simulink model "handsteuer_Joystick"  (Simulink 8.9)
settings: Solver=ode4  StartTime=0.0  StopTime=1200  FixedStep=0.01  RelTol=1e-3  EnableMultiTasking=on
undefined symbols (not defined in the file or in its folder): Joystick, National_Instruments, PCIe, Standard_Devices
libraries: sldrtlib x3, cstblocks x1
CloseFcn:
  | rtwprivate ssgencode ModelCloseRequest handsteuer_Joystick
settings Model: Creator=Praktikum  LastModifiedBy=prt01  SimulationMode=external  ExtModeTrigDuration=1000000
settings OptimizationCC: ExpressionDepthLimit=2147483647  InitFltsAndDblsToZero=on  LifeSpan=auto
settings DebuggingCC: SaveWithParameterizedLinksMsg=none  SignalResolutionControl=TryResolveAllWithWarning  SolverPrmCheckMsg=warning  MultiTaskDSMMsg=warning  MultiTaskCondExecSysMsg=none
settings HardwareCC: ProdBitPerPointer=64  ProdBitPerSizeT=64  ProdBitPerPtrDiffT=64  ProdLargestAtomicFloat=Float  ProdIntDivRoundTo=Zero  ProdEndianess=LittleEndian  ProdWordSize=64  ProdHWDeviceType=Intel->x86-64 (Windows64)
settings RTWCC: SystemTargetFile=sldrt.tlc  TemplateMakefile=sldrt.tmf  Description=Simulink Desktop Real-Time  RTWCompilerOptimization=on
settings CodeAppCC: MaxIdLength=95
settings SimulinkDesktopRealTimeCC: TargetFcnLib=ansi_tfl_tmw.mat  TargetPreCompLibLocation=C:\Program Files\MATLAB\R2017a\toolbox\sldrt\lib\win64  TargetLangStandard=C89/C90 (ANSI)  ModelReferenceCompliant=off  CompOptLevelCompliant=off  SupportVariableSizeSignals=off

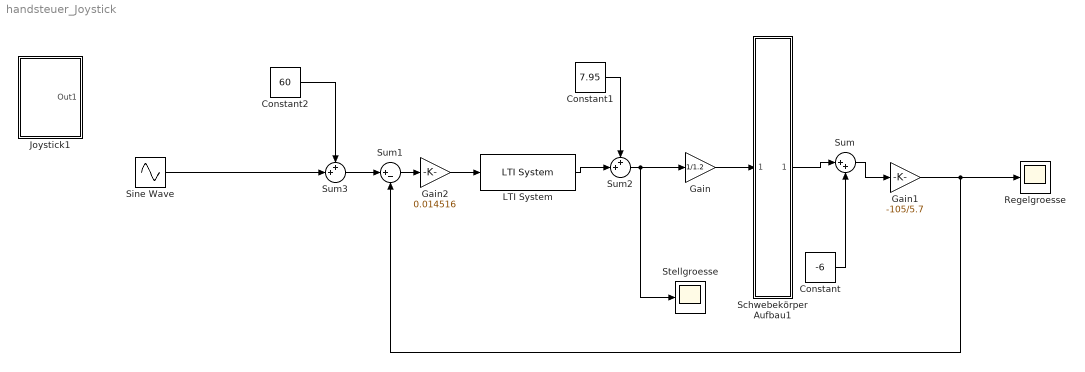
== system handsteuer_Joystick ==
  Constant : Constant  Value=-6
  Constant1 : Constant  Value=7.95
  Constant2 : Constant  Value=60
  Gain : Gain  Gain=1/1.2
  Gain1 : Gain  Gain=-105/5.7
  Gain2 : Gain  Gain=0.014516
  Joystick1 : Subsystem
      mask Display: image(imread('Joystick.bmp'))
  LTI System : cstblocks/LTI System  sys=tf([0.84 2.5 1],[0.05 1 0])  IC=[]
  Regelgroesse : Scope
  Schwebekörper Aufbau1 : Subsystem
      mask Display: image(imread('SKAufbauSkizze1.jpg'))
  Sine Wave : Sin  Amplitude=20  SampleTime=0
  Stellgroesse : Scope
  Sum : Sum  Inputs=|++
  Sum1 : Sum  Inputs=|+-
  Sum2 : Sum  Inputs=++|
  Sum3 : Sum  Inputs=++|
  wires:
  Gain/1 -> Schwebekörper Aufbau1/1(uDA)
  Gain1/1 -> Regelgroesse/1, Sum1/2
  Constant/1 -> Sum/2
  Schwebekörper Aufbau1/1(yAD) -> Sum/1
  Sum/1 -> Gain1/1
  Sum1/1 -> Gain2/1
  LTI System/1 -> Sum2/2
  Constant1/1 -> Sum2/1
  Sum2/1 -> Stellgroesse/1, Gain/1
  Constant2/1 -> Sum3/1
  Sum3/1 -> Sum1/1
  Gain2/1 -> LTI System/1
  Sine Wave/1 -> Sum3/2

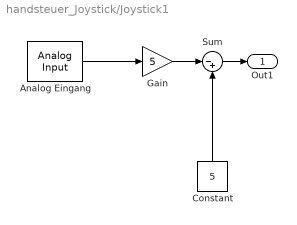
== system handsteuer_Joystick/Joystick1 ==
  Analog Eingang : sldrtlib/Analog Input  SampleTime=0.01  MaxMissedTicks=10  ShowMissedTicks=off  YieldWhenWaiting=off  DrvName=Standard_Devices/Joystick  DrvAddress=1  DrvOptions=zeros(1,0)  Channels=2  RangeMode=1  VoltRange=1  DataType=1
      settings: AttributesFormatString=Standard Devices\nJoystick [1h]  SourceProductName=Simulink Desktop Real-Time
  Constant : Constant  Value=5
  Gain : Gain  Gain=5
  Sum : Sum  Inputs=|-+
  Out1 : Outport
  wires:
  Sum/1 -> Out1/1
  Constant/1 -> Sum/2
  Gain/1 -> Sum/1
  Analog Eingang/1 -> Gain/1

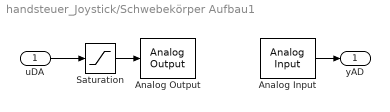
== system handsteuer_Joystick/Schwebekörper Aufbau1 ==
  uDA : Inport
  Analog Input : sldrtlib/Analog Input  SampleTime=0.01  MaxMissedTicks=10  ShowMissedTicks=off  YieldWhenWaiting=off  DrvName=National_Instruments/PCIe-6321  DrvAddress=4294967295  DrvOptions=[0 0 0 0 0 0 0]  Channels=1  RangeMode=1  VoltRange=1  DataType=1
      settings: AttributesFormatString=National Instruments\nPCIe-6321 [auto]  SourceProductName=Simulink Desktop Real-Time
  Analog Output : sldrtlib/Analog Output  SampleTime=0.01  MaxMissedTicks=10  ShowMissedTicks=off  YieldWhenWaiting=off  DrvName=National_Instruments/PCIe-6321  DrvAddress=4294967295  DrvOptions=[0 0 0 0 0 0 0]  Channels=1  RangeMode=1  VoltRange=1  InitialValue=0  FinalValue=0
      settings: AttributesFormatString=National Instruments\nPCIe-6321 [auto]  SourceProductName=Simulink Desktop Real-Time
  Saturation : Saturate  UpperLimit=10  LowerLimit=0
  yAD : Outport
  wires:
  Analog Input/1 -> yAD/1
  uDA/1 -> Saturation/1
  Saturation/1 -> Analog Output/1
